simulink model "object_detection"  (R2022a)
settings: Solver=ode4  StartTime=0.0  StopTime=inf  FixedStep=1/30  RelTol=1e-3  EnableMultiTasking=on
undefined symbols (not defined in the file): height, left, qc_get_step_size, top, Video3D, width
libraries: quarc_library x19, simulink x1
settings Model: SimulationMode=external  ExtModeTrigDuration=10000  Creator=fvranes  LastModifiedBy=mbohra
settings SolverCC: AlgebraicLoopSolver=TrustRegion  PositivePriorityOrder=on
settings DataIOCC: SaveOutput=off  SignalLogging=off  DSMLogging=off  SaveTime=off  ReturnWorkspaceOutputs=off
settings DebuggingCC: UnconnectedInputMsg=warning  UnconnectedOutputMsg=warning  UnconnectedLineMsg=warning  ArithmeticOperatorsInVariantConditions=warning
settings SFSimCC: SimUseLocalCustomCode=off  CustomCodeUndefinedFunction=UseInterfaceOnly
settings RTWCC: Description=QUARC Win64 Target Using Toolchain  SystemTargetFile=quarc_win64.tlc  TemplateMakefile=quarc_default_tmf  RTWUseLocalCustomCode=off  Toolchain=QUARC win64 | nmake (64-bit Windows)  BuildConfiguration=Faster Runs  DLArmComputeVersion=19.05
settings CodeAppCC: StateflowObjectComments=on
settings STFCustomTargetCC: TargetLangStandard=C99 (ISO)  ConcurrentExecutionCompliant=on  UseToolchainInfoCompliant=on  SystemTargetFile=quarc_win64.tlc
settings GRTTargetCC: ParMdlRefBuildCompliant=off  CompOptLevelCompliant=off  CombineOutputUpdateFcns=off  MatFileLogging=off  CPPClassGenCompliant=off  GRTInterface=on  ExtMode=on  ExtModeMexFile=quarc_comm
settings ConfigComp: CovMetricSettings=dswe

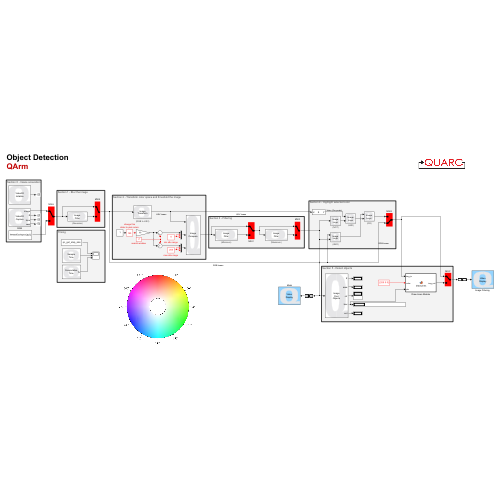
[thumbnail: Simulink's stored preview of the top-level diagram]
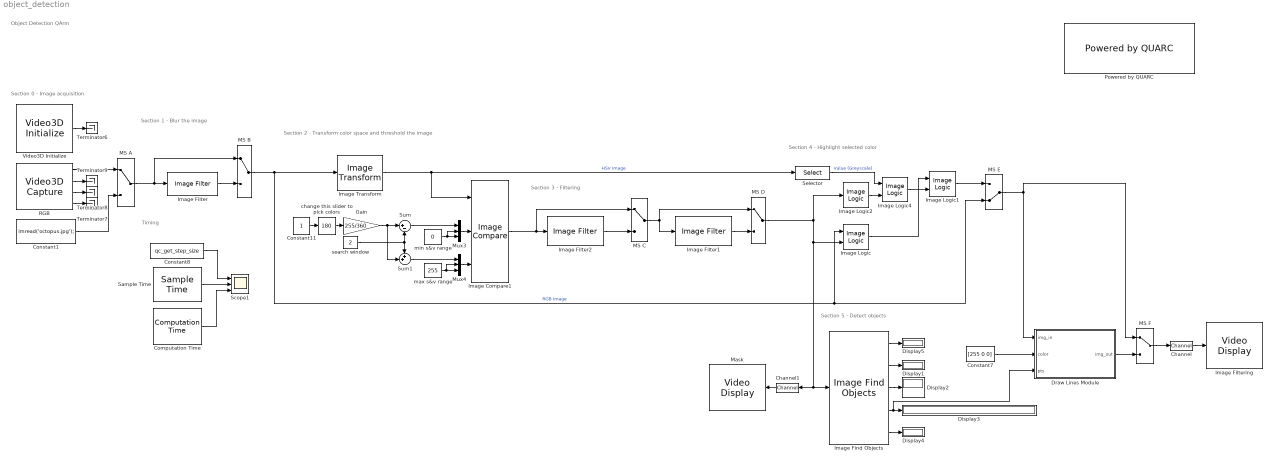
== system object_detection ==
  note: Section 4 - Highlight selected color
  note: Section 3 - Filtering
  note: Section 2 - Transform color space and threshold the image
  note: Section 1 - Blur the image
  note: Timing
  note: Object Detection
      | QArm
  note: Section 5 - Detect objects
  note: Section 0 - Image acquisition
  Channel : quarc_library/Signal Routing/Channel  channel=0  buffer_size=1
  Channel1 : quarc_library/Signal Routing/Channel  channel=1  buffer_size=1
  Computation Time : quarc_library/Sources/Time/Computation Time  sample_time=qc_get_step_size  use_model=on  use_cpu_time=off
  Constant1 : Constant  Value=imread('octopus.jpg');
  Constant11 : Constant
  Constant7 : Constant  Value=[255 0 0]
  Constant8 : Constant  Value=qc_get_step_size
  Display{1..5} (5 alike) : Display
  Draw Lines Module : MATLAB Function  TreatAsAtomicUnit=on
  Gain : Gain  Gain=255/360
  Image Compare1 : quarc_library/Image Processing/Generic/Image Compare  output_type=Combined (one HxW output)  source=External input ports  r_comparison=min <= pixel and pixel <= max with wrapping  r_minimum=0  r_maximum=10  g_comparison=min <= pixel and pixel <= max with wrapping  g_minimum=0  g_maximum=64  b_comparison=min <= pixel and pixel <= max with wrapping  b_minimum=0  b_maximum=200
      settings: SourceProductName=QUARC Targets
  Image Filter : quarc_library/Image Processing/Generic/Image Filter  filter_type=Gaussian  source_of_roi=Internal dialog parameter  roi_style=[top, left, height, width]  roi=[]  maximum_roi=[]  roi_zone=Operate inside region of interest  border_type=Replicate  border_value=[0 0 0]  kernel_size=5  sigma=1  mask_size=[3 3]  kernel=int16([-2 -1 0; -1 1 1; 0 1 2])  divisor=1  offset=0  rounding=Nearest  algorithm_hint=None  threshold=100  alpha=0.9  num_frames=8  num_valid=1  gap_threshold=10  depth_threshold=255  iterations=2
      settings: AttributesFormatString=(%<filter_type>)  SourceProductName=QUARC Targets
  Image Filter1 : quarc_library/Image Processing/Generic/Image Filter  filter_type=Maximum  source_of_roi=Internal dialog parameter  roi_style=[top, left, height, width]  roi=[]  maximum_roi=[]  roi_zone=Operate inside region of interest  border_type=Replicate  border_value=[0 0 0]  kernel_size=15  sigma=.2  mask_size=[5 5]  kernel=int16([-2 -1 0; -1 1 1; 0 1 2])  divisor=1  offset=0  rounding=Nearest  algorithm_hint=None  threshold=100  alpha=0.9  num_frames=8  num_valid=1  gap_threshold=10  depth_threshold=255  iterations=2
      settings: AttributesFormatString=(%<filter_type>)  SourceProductName=QUARC Targets
  Image Filter2 : quarc_library/Image Processing/Generic/Image Filter  filter_type=Minimum  source_of_roi=Internal dialog parameter  roi_style=[top, left, height, width]  roi=[]  maximum_roi=[]  roi_zone=Operate inside region of interest  border_type=Replicate  border_value=[0 0 0]  kernel_size=15  sigma=.2  mask_size=[5 5]  kernel=int16([-2 -1 0; -1 1 1; 0 1 2])  divisor=1  offset=0  rounding=Nearest  algorithm_hint=None  threshold=100  alpha=0.9  num_frames=8  num_valid=1  gap_threshold=10  depth_threshold=255  iterations=2
      settings: AttributesFormatString=(%<filter_type>)  SourceProductName=QUARC Targets
  "Image Filtering " : quarc_library/Multimedia/Video Display  Tag=object_detection_/Image Filtering  sample_time=-1  use_hardware=on
  Image Find Objects : quarc_library/Image Processing/Generic/Image Find Objects  num_objects=1  connectivity=8 directions (N, NE, E, SE, S, SW, W, NW)  sort_order=Sort by number of pixels  min_pixels=10  max_pixels=intmax('uint32')  largest=on  exclude_at_edges=off  variable_size=off  use_complex=off
      settings: SourceProductName=QUARC Targets
  Image Logic : quarc_library/Image Processing/Generic/Image Logic  algorithm=AND  source=Internal dialog parameter  row=0  column=0
      settings: AttributesFormatString=(%<algorithm>)  SourceProductName=QUARC Targets
  Image Logic1 : quarc_library/Image Processing/Generic/Image Logic  algorithm=OR  source=Internal dialog parameter  row=0  column=0
      settings: AttributesFormatString=(%<algorithm>)  SourceProductName=QUARC Targets
  Image Logic2 : quarc_library/Image Processing/Generic/Image Logic  algorithm=NOT  source=Internal dialog parameter  row=0  column=0
      settings: AttributesFormatString=(%<algorithm>)  SourceProductName=QUARC Targets
  Image Logic4 : quarc_library/Image Processing/Generic/Image Logic  algorithm=AND  source=Internal dialog parameter  row=0  column=0
      settings: AttributesFormatString=(%<algorithm>)  SourceProductName=QUARC Targets
  Image Transform : quarc_library/Image Processing/Generic/Image Transform  algorithm=RGB to HSV  color_theme=KRYGCBMW  min_pixel=0  max_pixel=4000  focal_length=308  principal_point=[262 334]  radial_coeffs=[-0.3129 0.0907]  tangential_coeffs=[]  extrapolated_pixel=0  interpolation=nearest  row_coords=0  column_coords=0  output_height=480  output_width=640  angle=0  origin=[240 320]  output_origin=[240 320]  output_data_type=uint8
      settings: AttributesFormatString=(%<algorithm>)  SourceProductName=QUARC Targets
  MS A : ManualSwitch
  MS B : ManualSwitch
  MS C : ManualSwitch
  MS D : ManualSwitch
  MS E : ManualSwitch  CurrentSetting=0
  MS F : ManualSwitch
  Mask : quarc_library/Multimedia/Video Display  Tag=object_detection_/Mask  sample_time=-1  use_hardware=on
  Mux3 : Mux  Inputs=3
  Mux4 : Mux  Inputs=3
  Powered by QUARC : quarc_library/Logos/Powered by QUARC
  RGB : quarc_library/Multimedia/Video3D Capture  object_name=unassigned  stream_type=RGB  stream_index=0  resolution=640 x 480  width=640  height=480  output_format=MATLAB RGB (HxWx3)  data_type=uint8  sample_time=qc_get_step_size  camera_intrinsics=off  depth_scale=off  brightness_override=off  brightness=50.0  contrast_override=off  contrast=50.0  hue_override=off  hue=50.0  saturation_override=off  saturation=50.0  sharpness_override=off  sharpness=50.0  gamma_override=off  gamma=50.0  gain_override=off  gain=50.0  backlightcompensation_override=off  backlightcompensation=50.0  whitebalance_override=Automatic white balance  whitebalance=50.0  exposure_override=Automatic exposure  exposure=30.0  emitter=Enable laser emitter  preset=Do not set camera presets
  Sample Time : quarc_library/Sources/Time/Sample Time  Priority=-99  sample_time=qc_get_step_size
  Scope1 : Scope  NumInputPorts=3
  Selector : Selector  NumberOfDimensions=3  InputPortWidth=3  IndexOptions=Select all,Select all,Index vector (dialog)  Indices=[1 3],1,3  OutputSizes=1,1,1
  Sum : Sum  Inputs=|+-
  Sum1 : Sum  Inputs=++|
  Terminator{6..9} (4 alike) : Terminator
  Video3D Initialize : quarc_library/Multimedia/Video3D Initialize  object_name=Video3D-1  source=Device  identifier=0  file=sample.bag  sample_time=qc_get_step_size  active=on
  change this slider to pick colors : simulink/Math Operations/Slider Gain  gain=180  low=0  high=360
  max s&v range : Constant  Value=255
  min s&v range : Constant  Value=0
  search window : Constant  Value=2
  wires:
  Sample Time/1 -> Scope1/2
  Image Compare1/1 -> MS C/1, Image Filter2/1
  Image Find Objects/1 -> Display5/1
  Image Find Objects/2 -> Display1/1
  Image Find Objects/3 -> Display2/1
  Image Find Objects/4 -> Draw Lines Module/3(pts), Display3/1
  Constant7/1 -> Draw Lines Module/2(color)
  Image Transform/1 -> Image Compare1/1, Selector/1  "HSV Image"
  Image Find Objects/5 -> Display4/1
  Image Filter1/1 -> MS D/2
  MS E/1 -> MS F/1, Draw Lines Module/1(img_in)
  Constant8/1 -> Scope1/1
  Computation Time/1 -> Scope1/3
  Mux3/1 -> Image Compare1/2
  Mux4/1 -> Image Compare1/3
  Sum1/1 -> Mux4/1
  Gain/1 -> Sum/1, Sum1/2
  change this slider to pick colors/1 -> Gain/1
  min s&v range/1 -> Mux3/3, Mux3/2
  Sum/1 -> Mux3/1
  max s&v range/1 -> Mux4/2, Mux4/3
  Constant11/1 -> change this slider to pick colors/1
  Draw Lines Module/1(img_out) -> MS F/2
  Channel/1 -> "Image Filtering "/1
  MS F/1 -> Channel/1
  Image Logic1/1 -> MS E/1
  Channel1/1 -> Mask/1
  Image Filter2/1 -> MS C/2
  MS C/1 -> Image Filter1/1, MS D/1
  Selector/1 -> Image Logic4/1  "Value (Greyscale)"
  Image Logic/1 -> Image Logic1/1
  MS B/1 -> Image Logic/1, MS E/2, Image Transform/1  "RGB Image"
  Image Logic2/1 -> Image Logic4/2
  search window/1 -> Sum1/1, Sum/2
  MS D/1 -> Image Logic/2, Channel1/1, Image Find Objects/1, Image Logic2/1
  Image Logic4/1 -> Image Logic1/2
  MS A/1 -> MS B/1, Image Filter/1
  Image Filter/1 -> MS B/2
  Constant1/1 -> MS A/2
  RGB/2 -> Terminator9/1
  RGB/3 -> Terminator8/1
  RGB/4 -> Terminator7/1
  Video3D Initialize/1 -> Terminator6/1
  RGB/1 -> MS A/1

== matlab function object_detection/Draw Lines Module ==
  data: img_in input; color input; img_out output; pts input
function img_out = drawLines(img_in, color, pts)

% Draw lines connecting the points using the provided color

% Inputs:
% img_in    : Input RGB Image (size = m by n)
% color     : 1x3 matrix of RGB color values for each marker
% pts       : p x-y pairs of points (px) where markers are to be drawn

% Outputs:
% img_out   : Output RGB Image with the markers drawn in (size = m by n)

%% Initialization
if size(img_in, 3) == 3
    img_out = img_in;
elseif size(img_in, 3) == 1
    img_out = cat(3, img_in, img_in, img_in);
end

box = single(pts (:,1)); % data on the box of the largest object

pts = [box(1), box(2); box(1), box(4); box(3), box(4); box(3), box(2); box(1), box(2)];

%points = pts;

[p, ~] = size(pts); % determine the number of points

%% Draw the lines

    for i = 1:p-1
        % determine the max(rows_difference, col_difference) between two
        % points
        itr = ceil(max(abs(pts(i,1) - pts(i+1,1)), abs(pts(i,2) - pts(i+1,2))));
        
        % generate linear spaces of row and col values between the pts
        row_vec = round(linspace(pts(i,1), pts(i+1,1), itr));
        col_vec = round(linspace(pts(i,2), pts(i+1,2), itr));
        
        % iterate through the values and shade them right

        for j = 1:itr
            img_out(row_vec(j), col_vec(j),1) = color(1);
            img_out(row_vec(j), col_vec(j),2) = color(2);
            img_out(row_vec(j), col_vec(j),3) = color(3);
        end
    end
end
